simulink model "Latest_Greatest"  (Simulink 10.1)
settings: Solver=ode4  StartTime=0  StopTime=15  FixedStep=DeltaT  RelTol=1e-3  EnableMultiTasking=on
InitFcn:
  | % Bifocal Relay Mirror Spacecraft (prior to payload installation) Dynamics Simulation          TA Sands
  | clear all;close all;clc;warning off all;
  | 
  | % Simulation run parameters
  | Rate=1000;  DeltaT=1/Rate;
  | 
  | % Maneuver Parameters
  | roll=0;  pitch=0; yaw=60;   roll=roll*pi/180; pitch=pitch*pi/180; yaw=yaw*pi/180;
  | SlewTime=5;   SACengage=0;
  | 
  | %Constants0
  | Re=6371.2e3;mu=398601.2e9;          %earth radius and universal gravitation constant
  | 
  | %Spacecraft orbit
  | h=0;                                     %orbit altitude
  | R=Re+h;                             %orbit radius from center of earth
  | we=0.000072921158553;   %earth's angular velocity rad/solar sec(Vallado)
  | wo=sqrt(mu/(Re+h)^3);        %orbit angular velocity
  | incln=36.6001*pi/180;          %Inclination assumed Monterey Latitude
  | epsilon=12*pi/180;  alphao=0;
  | uo=0; nuo=0;                        %Start S/C beneath subsolar point
  | beta=60; gamma=1.5;
  | a=0.545491852; b=0.314939867;  c=0.704226952;   %Assumed spacecraft rectangular size
  | Area=[b*c a*c a*b];                 %projected area~m^2 in body x,y,z directions
  | density=4.39e-14;
  | kpre=-9.9639/24/3600/180*pi*0;      %nodal precession constant assumed zero here
  | wn=kpre*(Re/(Re+h))^3.5*cos(incln); %nodal precession (zero eccentricity)
  | V=wo*(Re+h);
  | rho=asin(Re/(h+Re));                %earth angular radius
  | Cd=2.5;     psun=4.5E-6;            %Drag coefficient and solar pressure constant~N/m^2
  | Kaero=-0.5*Cd*V^2;   Psolar=2*psun;  %constants for aero and solar torque calculation
  | dL=[0.002 0.002 0.008];             %predicted distance between cp and cg
  | Kme=2.3390e-005;
  | 
  | %Spacecraft Magnetic Properties (assumed)
  | mresid=[0 0 0.01];                  %Spacecraft residual magnetic moment
  | M=mresid;                           %Magnetic unit dipole vector
  | K=7.943e15;
  | 
  | % ACTUAL Spacecraft Inertia conditions
  | Ix=90;   Iy=100;   Iz=250 ;
  | Ixy=-10;  Iyz=20;  Ixz=-10;
  | Imo=[Ix -Ixy -Ixz;
  |        -Ixy  Iy  -Iyz;
  |        -Ixz -Iyz  Iz];                  %Moment of inertia matrix
  | Iinv=inv(Imo);                      %Moment of inertia inverse goes in dynamics block
  | 
  | %Spacecraft initial Euler state angles and rates
  | phio=0;thetao=0;psio=0;                    %Initial Euler Angles
  | phidoto=0;thetadoto=0;psidoto=0;     %Initial Euler Rates
  | 
  | %Calculation of initial quaternion (qo) and angular momentum (Ho)
  | s1=sin(phio/2);s2=sin(thetao/2);s3=sin(psio/2);c1=cos(phio/2);c2=cos(thetao/2);c3=cos(psio/2);
  | q1o=s1*c2*c3-c1*s2*s3;
  | q2o=c1*s2*c3+s1*c2*s3;              %Wie pg. 321
  | q3o=c1*c2*s3-s1*s2*c3;
  | q4o=c1*c2*c3+s1*s2*s3;
  | S1=sin(phio);S2=sin(thetao);S3=sin(psio);C1=cos(phio);C2=cos(thetao);C3=cos(psio);
  | wxo=phidoto-psidoto*S2-wo*S3*C2;
  | wyo=thetadoto*C1+psidoto*C2*S1-wo*(C3*C1+S3*S2*S1);
  | wzo=psidoto*C2*C1-thetadoto*S1-wo*(S3*S2*C1-C3*S1);
  | qo=[q1o q2o q3o q4o];
  | Ho=Imo*[wxo wyo wzo]';
  | norm(Ho)*1000;
  | 
  | %Calculate eclipse time for comparison with EPS calculations
  | Te=100.87*2*V/2/pi;
  | 
  | %CMG Properties (in degrees)
  | %beta=90*pi/180;                                     %Skew angle in degrees converted to radians
  | beta=[90;90;-90;0]; beta=beta.*pi./180;
  | %beta=[54.73;54.73;-54.73;0]; beta=beta.*pi./180;
  | 
  | Gimbal0=[-30*pi/180; 90*pi/180; -30*pi/180;0];   % Initial Gimbal angles for 0 H spin up
  | w_wheel=2800*(2*pi/60);                       %Wheel speed in RPM converted to rad/s
  | Iwheel=0.0614*1.3558179483314;        % Wheel inertia in slug-ft^2 converted (exact) to kg m^2
  | h_wheel=Iwheel*w_wheel;                     % CMG Wheel Angular Momentum
  | 
  | %FEEDFORWARD (ASSUMED) Spacecraft Inertia conditions
  | Ix=119.1259;   Iy=150.6615;   Iz=106.0288;   %ACTUAL Values are Ix=90;   Iy=100;   Iz=250 ;
  | Ixy=-15.7678;  Iyz=22.31637;  Ixz=-6.54859;  %ACTUAL Values are Ixy=-10;  Iyz=20;  Ixz=-10;
  | Imo=[Ix -Ixy -Ixz;
  |        -Ixy  Iy  -Iyz;
  |        -Ixz -Iyz  Iz];                  %Moment of inertia matrix
  | THETAo=[Ix Ixy Ixz Iy Iyz Iz 0 0 0];
  | 
  | % [Fossen]'s adaptive feedforward parameters
  | ETA=1;LAMBDA=0;  uffGain=1;
  | 
  | %FEEDBACK CONTROLLERS Follow
  | %PDI Controller Gains  % TUNED Well for Presence of LOWPASS (Kp=0.5; Kd=Kp*750;  Ki=0.1)
  | %Kp=0.5;  Kd=Kp*750;  Ki=0.1;
  | 
  | %PDI Controller Gains  % TUNED WELL FOR NO-NOISE (Kp=1; Kd=2000*Kp; Ki=5)
  | Kp=1;   Kd=Kp*6000;    Ki=5;
  | 
  | %PDI Controller Gains  % TUNED WELL FOR NOISE (Kp=1; Kd=Kp*3000; Ki=1)
  | %Kp=1;   %Kd=Kp*3000;   %Ki=1;
  | 
  | %PID Controller Gains tuned well for uff and ufb decoupling
  | Kpx=20;  Kdx=1000;  Kix=0.1;
  | 
  | %Bandpass filter pole per Bong Wie 2nd Edition pg 137-138
  | wp=10*pi/SlewTime;       % Product of pole frequency and zero frequency establishes max phase lag
  | wz=2*wp;
  | dampZ=1;  % >0 but small for good tracking..
  | dampP=dampZ;
  | % Sensor Noise Parameters
  | NoiseVariance=1e-9;             BADNoiseVariance=NoiseVariance*1e3;
  | 
  | % Observer Gains
  | MaxI=300;  lambda1=12.5  ;   lambda2=50 ;   lambda3= 200;
  | Kdo=MaxI*(lambda1+lambda2+lambda3)/10;
  | Kpo=MaxI*(lambda1*(lambda2+lambda3)+lambda2*lambda3)/10;
  | Kio=MaxI*lambda1*lambda2*lambda3/9;
StopFcn:
  | if flag==0; Hcmg=Hcmg;else;Hcmg=HcmgMP;end;
  | Hxcmg=[];Hycmg=[];Hzcmg=[];CondA=[]; CondA_MP=[];t=[]; SingPt=[];DetA=[];
  | for i=1:max(size(A));  t=[t i*DeltaT];  H=Hcmg(:,:,i); Hx=H(1,:);  Hy=H(2,:);  Hz=H(3,:);
  | detA=det(A(:,1:3,i));Hxcmg=[Hxcmg Hx];  Hycmg=[Hycmg Hy];  Hzcmg=[Hzcmg Hz];
  | CONDA=cond(A(:,:,i));
  | DetA=[DetA detA]; DetA=1./DetA;
  | CondA=[CondA CONDA];end;   %CondA=CondA./max(CondA); DetA=DetA./max(DetA);
  | Hmag=sqrt(Hxcmg.^2+Hycmg.^2+Hzcmg.^2);x=(max(t)-DeltaT);
  | 
  | InvCondA;
  | 
  | if flag==0; MaxInvCond=min(1./CondA(10*Rate+1:end));DELTA=delta;DELTAdot=deltadot;
  | else; MaxInvCond=min(1./CondA_MP(10*Rate+1:end));DELTA=delta_MP;DELTAdot=deltadot_MP;Hcmg=HcmgMP;end;
  | 
  | ERROR=(trajectory*180/pi-Euler);
  | 
  | figure(1); wdotTrajectory=[CMDTrajectory(:,1) CMDTrajectory(:,2) CMDTrajectory(:,3)];  wTrajectory=[CMDTrajectory(:,4) CMDTrajectory(:,5) CMDTrajectory(:,6)]; ThetaTrajectory=180/pi.*[trajectory(:,1) trajectory(:,2) trajectory(:,3)];
  | subplot(3,1,1); plot(t,wdotTrajectory,'linewidth',2); axis tight; grid; ylabel('\omega^d^o^t_C_M_D (deg)','fontsize',16); title('Desired Angle, Rate, Acceleration Trajectories','fontsize',16);   set(gca,'XTick',0:2:15);     set(gca,'XTickLabel',{' ',' ',' ',' ',' ',' ',' ',' ','15'});
  | subplot(3,1,2); plot(t,wTrajectory,'linewidth',2); axis tight; grid; ylabel('\omega_C_M_D (deg)','fontsize',16);set(gca,'XTick',0:2:15);     set(gca,'XTickLabel',{' ',' ',' ',' ',' ',' ',' ',' ','15'});
  | subplot(3,1,3); plot(t,ThetaTrajectory,'linewidth',2); axis tight; grid; ylabel('\theta_C_M_D (deg)','fontsize',16); xlabel('time (sec)','fontsize',16);
  | 
  | figure(2);
  | subplot(2,1,1);plot(t,Hmag,'LineWidth',3);   ylabel('|H_c_m_g|','Fontsize',16);grid;axis([0,x,0,3]); set(gca,'fontsize',16);set(gca,'XTickLabel',{' ',' ',' ',' ',' ',' ',' ',' ','15'});
  | subplot(2,1,2);plot(t,InvCondA,'linewidth',3);grid;xlabel('t(sec)','fontsize',14,'fontname','times');ylabel('Cond[A]','fontsize',14,'fontname','times');axis([0,max(t),0,21.82]); set(gca,'fontsize',16);
  | 
  | DELTA1=DELTA(1,:);DELTA2=DELTA(2,:);DELTA3=DELTA(3,:);DELTA4=DELTA(4,:);
  | DELTAdot1=DELTAdot(1,:);DELTAdot2=DELTAdot(2,:);DELTAdot3=DELTAdot(3,:);DELTAdot4=DELTAdot(4,:);
  | 
  | figure(3);subplot(4,1,1);plot(t,DELTA1,'LineWidth',3); title('Gimbal Angles','fontsize',16);ylabel('\theta_1(deg)','Fontsize',14);grid;axis tight; set(gca,'XTickLabel',{' ',' ',' ',' ',' ',' ',' ',' ','15'});set(gca,'fontsize',16);
  | subplot(4,1,2);plot(t,DELTA2,'LineWidth',3); ylabel('\theta_2(deg)','Fontsize',16);grid;axis tight; set(gca,'XTickLabel',{' ',' ',' ',' ',' ',' ',' ',' ','15'});set(gca,'fontsize',16);
  | subplot(4,1,3);plot(t,DELTA3,'LineWidth',3); ylabel('\theta_3(deg)','Fontsize',16);grid;axis tight; set(gca,'XTickLabel',{' ',' ',' ',' ',' ',' ',' ',' ','15'});set(gca,'fontsize',16);
  | subplot(4,1,4);plot(t,InvCondA,'linewidth',3);grid;xlabel('t(sec)','fontsize',14,'fontname','times');ylabel('Cond[A]','fontsize',14,'fontname','times');axis([0,max(t),0,21.82]); set(gca,'fontsize',16);
  | 
  | figure(4);subplot(4,1,1);plot(t,DELTAdot1,'LineWidth',3);  title('Gimbal Angle RATES','fontsize',16); ylabel('\theta_d_o_t_1(rad/s)','Fontsize',16);grid; axis([0,x,-pi*1.1,pi*1.1]);   set(gca,'XTickLabel',{' ',' ',' ',' ',' ',' ',' ',' ','15'});set(gca,'fontsize',16);
  | subplot(4,1,2);plot(t,DELTAdot2,'LineWidth',3);   ylabel('\theta_d_o_t_2(rad/s)','Fontsize',16);grid;axis([0,x,-pi*1.1,pi*1.1]);   set(gca,'XTickLabel',{' ',' ',' ',' ',' ',' ',' ',' ','15'});   set(gca,'fontsize',16);
  | subplot(4,1,3);plot(t,DELTAdot3,'LineWidth',3);   ylabel('\theta_d_o_t_3(rad/s)','Fontsize',16);grid;axis([0,x,-pi*1.1,pi*1.1]); set(gca,'XTickLabel',{' ',' ',' ',' ',' ',' ',' ',' ','15'});set(gca,'fontsize',16);
  | subplot(4,1,4);plot(t,InvCondA,'linewidth',3);grid;xlabel('t(sec)','fontsize',14,'fontname','times');ylabel('Cond[A]','fontsize',14,'fontname','times');axis([0,max(t),0,21.82]); set(gca,'fontsize',16);
  | 
  | figure(5);
  | subplot(4,1,1);plot(t,Hxcmg,'linewidth',3);axis([0,x,-3.25,3.25]);grid;ylabel('h_x/|h|','fontsize',16);title('Normalized Momentum','fontsize',16);set(gca,'XTickLabel',{' ',' ',' ',' ',' ',' ',' ',' ','15'});set(gca,'fontsize',16);
  | subplot(4,1,2);plot(t,Hycmg,'linewidth',3);axis([0,x,-3.25,3.25]);grid;ylabel('h_y/|h|','fontsize',16);set(gca,'XTickLabel',{' ',' ',' ',' ',' ',' ',' ',' ','15'});set(gca,'fontsize',16);
  | subplot(4,1,3);plot(t,Hzcmg,'linewidth',3);axis([0,x,-3.25,3.25]);grid;ylabel('h_z/|h|','fontsize',16);  set(gca,'XTickLabel',{' ',' ',' ',' ',' ',' ',' ',' ','15'});set(gca,'fontsize',16);
  | subplot(4,1,4);plot(t,InvCondA,'linewidth',3);grid;xlabel('t(sec)','fontsize',14,'fontname','times');ylabel('Cond[A]','fontsize',14,'fontname','times');axis([0,max(t),0,21.82]); set(gca,'fontsize',16);
  | 
  | figure(6); EulerX=Euler(:,1);EulerY=Euler(:,2);EulerZ=Euler(:,3);
  | subplot(4,1,1);plot(t,EulerX,'linewidth',3); axis([0,x,min(EulerX)*5,max(EulerX)*5]);grid;ylabel('\phi(deg)','fontsize',16);title('True Euler Angles','fontsize',14);  set(gca,'XTickLabel',{' ',' ',' ',' ',' ',' ',' ',' ','15'});  set(gca,'fontsize',16);
  | subplot(4,1,2);plot(t,EulerY,'linewidth',3);  axis([0,x,min(EulerY)*5,max(EulerY)*5]); grid;ylabel('\theta(deg)','fontsize',14);  set(gca,'XTickLabel',{' ',' ',' ',' ',' ',' ',' ',' ','15'}); set(gca,'fontsize',16);
  | subplot(4,1,3);plot(t,EulerZ,'linewidth',3);axis([0,x,min(EulerZ)*1.25,max(EulerZ)*1.25]);grid;  ylabel('\psi(deg)','fontsize',14);  set(gca,'XTickLabel',{' ',' ',' ',' ',' ',' ',' ',' ','15'});  set(gca,'fontsize',16);
  | subplot(4,1,4);plot(t,InvCondA,'linewidth',3);grid;xlabel('t(sec)','fontsize',14,'fontname','times');ylabel('Cond[A]','fontsize',14,'fontname','times');axis([0,max(t),0,21.82]); set(gca,'fontsize',16);
  | 
  | EX=ERROR(:,1);  EY=ERROR(:,2);     EZ=ERROR(:,3);
  | MeanXerror=mean(EX); Xmean=num2str(MeanXerror); xmean=['\mu_\phi=', Xmean];
  | STDx=std(EX);Xsigma=num2str(STDx);SigmaX=['    \sigma_x=' Xsigma];  xlegend=[xmean, SigmaX];
  | MeanYerror=mean(EY); Ymean=num2str(MeanYerror); ymean=['\mu_\theta=', Ymean];
  | STDy=std(EY); Ysigma=num2str(STDy);SigmaY=['    \sigma_y=' Ysigma]; ylegend=[ymean, SigmaY];
  | MeanZerror=mean(EZ); Zmean=num2str(MeanZerror); zmean=['\mu_\psi=', Zmean];
  | STDz=std(EZ);Zsigma=num2str(STDz);SigmaZ=['    \sigma_z=' Zsigma]; zlegend=[zmean, SigmaZ];
  | MeanError=[MeanXerror MeanYerror MeanZerror];  StdDev=[STDx STDy STDz];
  | 
  | figure(7);
  | subplot(3,1,1);plot(t,EX,'linewidth',3);    axis([0,x,min(EX)*1.25,max(EX)*1.25]);  title('Euler Angle Tracking Error','fontsize',16);
  |      legend(xlegend, 'location','NorthEast');  grid   ; ylabel('\phi(deg)','fontsize',16);set(gca,'XTickLabel',{' ',' ',' ',' ',' ',' ',' ',' ','15'});set(gca,'fontsize',16);
  | subplot(3,1,2);plot(t,EY,'linewidth',3);   axis([0,x,min(EY)*1.25,max(EY)*1.25]);
  |       legend(ylegend, 'location','NorthEast');  grid;    ylabel('\theta(deg)','fontsize',16);set(gca,'XTickLabel',{' ',' ',' ',' ',' ',' ',' ',' ','15'});set(gca,'fontsize',16);
  | subplot(3,1,3);plot(t,EZ,'linewidth',3);    axis([0,x,min(EZ)*1.25,max(EZ)*1.25]);
  |      legend(zlegend, 'location','NorthEast');  grid;   ylabel('\psi(deg)','fontsize',16);xlabel('t(sec)','fontsize',16);set(gca,'fontsize',16);
  | 
  | figure(8);subplot(3,3,1);
  | plot(t,THETAhat(:,1),'linewidth',2);grid; axis tight;ylabel('J_x_x','fontsize',16);  set(gca,'XTickLabel',{' ',' ',' ',' ',' ',' ',' ',' ','15'});  set(gca,'fontsize',16);
  | subplot(3,3,2);plot(t,THETAhat(:,2),'linewidth',3);grid;axis tight;ylabel('J_x_y','fontsize',16);   set(gca,'XTickLabel',{' ',' ',' ',' ',' ',' ',' ',' ','15'});  set(gca,'fontsize',16);  title('Inertia & Momentum Adaption','fontsize',18);
  | subplot(3,3,3);plot(t,THETAhat(:,3),'linewidth',3);grid;axis tight;ylabel('J_x_z','fontsize',16);set(gca,'XTickLabel',{' ',' ',' ',' ',' ',' ',' ',' ','15'});set(gca,'fontsize',16);
  | subplot(3,3,4);plot(t,THETAhat(:,4),'linewidth',3);grid;axis tight;ylabel('J_y_y','fontsize',16);set(gca,'XTickLabel',{' ',' ',' ',' ',' ',' ',' ',' ','15'});set(gca,'fontsize',16);
  | subplot(3,3,5);plot(t,THETAhat(:,5),'linewidth',3);grid;axis tight;ylabel('J_y_z','fontsize',16);set(gca,'XTickLabel',{' ',' ',' ',' ',' ',' ',' ',' ','15'});set(gca,'fontsize',16);
  | subplot(3,3,6);plot(t,THETAhat(:,6),'linewidth',3);grid;axis tight;ylabel('J_z_z','fontsize',16);set(gca,'XTickLabel',{' ',' ',' ',' ',' ',' ',' ',' ','15'});set(gca,'fontsize',16);
  | subplot(3,3,7);plot(t,THETAhat(:,7),'linewidth',3);grid;axis tight;ylabel('H_x','fontsize',16);xlabel('t(sec)','fontsize',14);set(gca,'fontsize',16);
  | subplot(3,3,8);plot(t,THETAhat(:,8),'linewidth',3);grid;axis tight;ylabel('H_y','fontsize',16);xlabel('t(sec)','fontsize',14);set(gca,'fontsize',16);
  | subplot(3,3,9);plot(t,THETAhat(:,9),'linewidth',3);grid;axis tight;ylabel('H_z','fontsize',16);xlabel('t(sec)','fontsize',14);set(gca,'fontsize',16);
  | 
  | ControlX=sqrt(abs(ControlEffort(end,1)))/(max(t)); ControlStringX=num2str(ControlX); Control_x=['1/t sqrt(\int u^2_\phi dt)=', ControlStringX];
  | ControlY=sqrt(abs(ControlEffort(end,2)))/(max(t)); ControlStringY=num2str(ControlY); Control_y=['1/t sqrt(\int u^2_\theta dt)=', ControlStringY];
  | ControlZ=sqrt(abs(ControlEffort(end,3)))/(max(t)); ControlStringZ=num2str(ControlZ); Control_z=['1/t sqrt(\int u^2_\psi dt)=', ControlStringZ];
  | 
  | figure(9);
  | subplot(2,1,1);plot(t,ufb,'linewidth',3);grid; axis tight;ylabel('Feedback Control (Nm)','fontname','times','fontsize',14);  legend(Control_x, Control_y, Control_z, 'location','SouthEast');
  | title('Feedforward and Feedback Controls','fontsize',18);set(gca,'XTickLabel',{' ',' ',' ',' ',' ',' ',' ',' ','15'});set(gca,'fontsize',16);
  | subplot(2,1,2);plot(t,uff,'linewidth',3);grid; axis tight; ylabel('FeedForward Control (Nm)','fontname','times','fontsize',14);      xlabel('time(sec)','fontname','times','fontsize',14); set(gca,'fontsize',16);
  | 
  | figure(10);
  | subplot(4,1,1);plot(t,ufb(:,1),'linewidth',3);grid;ylabel('u_\phi(Nm)','fontsize',16);title('u_f_b (Nm)','fontsize',16); axis tight; set(gca,'XTickLabel',{' ',' ',' ',' ',' ',' ',' ',' ','15'});set(gca,'fontsize',16);
  | subplot(4,1,2);plot(t,ufb(:,2),'linewidth',3); grid;ylabel('u_\theta(Nm)','fontsize',16); axis tight; set(gca,'XTickLabel',{' ',' ',' ',' ',' ',' ',' ',' ','15'});set(gca,'fontsize',16);
  | subplot(4,1,3);plot(t,ufb(:,3),'linewidth',3); grid;ylabel('u_\psi(Nm)','fontsize',16); axis tight; set(gca,'XTickLabel',{' ',' ',' ',' ',' ',' ',' ',' ','15'});set(gca,'fontsize',16);
  | subplot(4,1,4);plot(t,InvCondA,'linewidth',3);grid;xlabel('t(sec)','fontsize',14,'fontname','times');ylabel('Cond[A]','fontsize',14,'fontname','times');axis([0,max(t),0,21.82]); set(gca,'fontsize',16);
  | 
  | % CALCULATE FIGURES OF MERIT FOR ESTIMATION ACCURACY OF LUENBERGER OBSERVER
  | EEX=EstimationError(:,1);EEY=EstimationError(:,2);EEZ=EstimationError(:,3);
  | MeanEEX=mean(EEX); EEXmean=num2str(MeanEEX); Exmean=['Luenberger \mu_\phi^o _E_r_r_o_r=', EEXmean];
  | MeanEEY=mean(EEY); EEYmean=num2str(MeanEEY); Eymean=['Luenberger \mu_\theta^o _E_r_r_o_r=', EEYmean];
  | MeanEEZ=mean(EEZ); EEZmean=num2str(MeanEEZ); Ezmean=['Luenberger \mu_\psi^o _E_r_r_o_r=', EEZmean];
  | STDEEX=std(EEX);                      EEXstd=num2str(STDEEX);         Exstd=['   \sigma_\phi^o _E_r_r_o_r=', EEXstd];
  | STDEEY=std(EEY);                      EEYstd=num2str(STDEEY);         Eystd=['   \sigma_\theta^o _E_r_r_o_r=', EEYstd];
  | STDEEZ=std(EEZ);                      EEZstd=num2str(STDEEZ);         Ezstd=['   \sigma_\psi^o _E_r_r_o_r=', EEZstd];
  | XlabelLuen=[Exmean Exstd];  YlabelLuen=[Eymean Eystd];  ZlabelLuen=[Ezmean Ezstd];
  | 
  | % CALCULATE FIGURES OF MERIT FOR ESTIMATION ACCURACY OF PID OBSERVERS
  | EEXo=PIDoEstimationError(:,1);EEYo=PIDoEstimationError(:,2);EEZo=PIDoEstimationError(:,3);
  | MeanEEXo=mean(EEXo); EEXmeano=num2str(MeanEEXo); Exmeano=['PID \mu_\phi^o _E_r_r_o_r=', EEXmeano];
  | MeanEEYo=mean(EEYo); EEYmeano=num2str(MeanEEYo); Eymeano=['PID \mu_\theta^o _E_r_r_o_r=', EEYmeano];
  | MeanEEZo=mean(EEZo); EEZmeano=num2str(MeanEEZo); Ezmeano=['PID \mu_\psi^o _E_r_r_o_r=', EEZmeano];
  | STDEEXo=std(EEXo);                      EEXstdo=num2str(STDEEXo);         Exstdo=['    \sigma_\phi^o _E_r_r_o_r=', EEXstdo];
  | STDEEYo=std(EEYo);                      EEYstdo=num2str(STDEEYo);         Eystdo=['    \sigma_\theta^o _E_r_r_o_r=', EEYstdo];
  | STDEEZo=std(EEZo);                      EEZstdo=num2str(STDEEZo);         Ezstdo=['    \sigma_\psi^o _E_r_r_o_r=', EEZstdo];
  | XlabelPID=[Exmeano Exstdo];  YlabelPID=[Eymeano Eystdo];  ZlabelPID=[Ezmeano Ezstdo];
  | 
  | % CALCULATE FIGURES OF MERIT FOR ESTIMATION ACCURACY OF KALMAN OBSERVERS
  | EEXkf=KalmanEstimationError(:,1);   EEYkf=KalmanEstimationError(:,2);        EEZkf=KalmanEstimationError(:,3);
  | MeanEEXkf=mean(EEXkf);                EEXmeankf=num2str(MeanEEXkf);         Exmeankf=['Kalman \mu_\phi^o _E_r_r_o_r=', EEXmeankf];
  | MeanEEYkf=mean(EEYkf);                EEYmeankf=num2str(MeanEEYkf);         Eymeankf=['Kalman \mu_\theta^o _E_r_r_o_r=', EEYmeankf];
  | MeanEEZkf=mean(EEZkf);                EEZmeankf=num2str(MeanEEZkf);         Ezmeankf=['Kalman \mu_\psi^o _E_r_r_o_r=', EEZmeankf];
  | STDEEXkf=std(EEXkf);                      EEXstdkf=num2str(STDEEXkf);         Exstdkf=['    \sigma_\phi^o _E_r_r_o_r=', EEXstdkf];
  | STDEEYkf=std(EEYkf);                      EEYstdkf=num2str(STDEEYkf);         Eystdkf=['    \sigma_\theta^o _E_r_r_o_r=', EEYstdkf];
  | STDEEZkf=std(EEZkf);                      EEZstdkf=num2str(STDEEZkf);         Ezstdkf=['    \sigma_\psi^o _E_r_r_o_r=', EEZstdkf];
  | Xlabelkf=[Exmeankf Exstdkf];  Ylabelkf=[Eymeankf Eystdkf];  Zlabelkf=[Ezmeankf Ezstdkf];
  | 
  | figure(11);
  | subplot(3,1,1);plot(t,KalmanEstimationError(:,1),'r:','linewidth',3); hold on; plot(t,PIDoEstimationError(:,1),'linewidth',3);  plot(t,EstimationError(:,1),'k--','linewidth',3);   set(gca,'fontsize',12);
  | ylabel('\phi Roll (deg)','fontsize',16);   title('Observer Estimation Error Comparison','fontsize',14);  legend(Xlabelkf,XlabelPID, XlabelLuen, 'location','NorthWest'); grid; axis([0,15,-0.01,0.04]);
  | set(gca,'XTickLabel',{' ',' ',' ',' ',' ',' ',' ',' ','15'});
  | 
  | subplot(3,1,2); plot(t,KalmanEstimationError(:,2),'r:','linewidth',3); hold on;  plot(t,PIDoEstimationError(:,2),'linewidth',3); plot(t,EstimationError(:,2),'k--','linewidth',3); set(gca,'fontsize',12);
  | ylabel('\theta Pitch (deg)','fontsize',16); hold off;  legend(Ylabelkf, YlabelPID, YlabelLuen, 'location','SouthWest'); grid;  set(gca,'XTickLabel',{' ',' ',' ',' ',' ',' ',' ',' ','15'});  axis([0,15,-0.08,0.03]);
  | 
  | subplot(3,1,3); plot(t,KalmanEstimationError(:,3),'r:','linewidth',3);  hold on;  plot(t,PIDoEstimationError(:,3),'linewidth',3);plot(t,EstimationError(:,3),'k--','linewidth',3);set(gca,'fontsize',12);
  | ylabel('\psi Yaw (deg)','fontsize',16);xlabel('t(sec)','fontsize',16);  hold off;  legend(Zlabelkf, ZlabelPID, ZlabelLuen,'location','NorthWest'); grid; axis tight;
  | 
  | %openfig('90_Degree_Singularity_Hypersurface');hold on;plot3(Hcmg(1,:),Hcmg(2,:),Hcmg(3,:), 'LineWidth',3);hold off;
  | 
  | QNORMSTD=std(qnorm);                      QNORMSTDSTRING=num2str(QNORMSTD);         QnormLEGEND=['    ||q||=', QNORMSTDSTRING];
  |  figure (12); plot(qnorm); legend([QnormLEGEND]);  grid;
undefined symbols (not defined in the file): magnitude, svd
libraries: aerospace x3, simulink_need_slupdate x2, dspadpt3 x2, dspinverses x1
(part 1 of 2)
settings Model: Creator=tasands  LastModifiedBy=Cornell Gaming Lapto
settings DataIOCC: LimitDataPoints=on  SignalLoggingSaveFormat=ModelDataLogs  SignalLoggingName=sigsOut
settings OptimizationCC: ExpressionDepthLimit=2147483647  InitFltsAndDblsToZero=on
settings DebuggingCC: SaveWithParameterizedLinksMsg=none  SignalResolutionControl=TryResolveAllWithWarning  MultiTaskDSMMsg=warning  MultiTaskCondExecSysMsg=none  FcnCallInpInsideContextMsg=warning  StateNameClashWarn=warning  PregeneratedLibrarySubsystemCodeDiagnostic=none
settings HardwareCC: TargetHWDeviceType=32-bit Generic  ProdEqTarget=off
settings GRTTargetCC: TargetFcnLib=ansi_tfl_tmw.mat

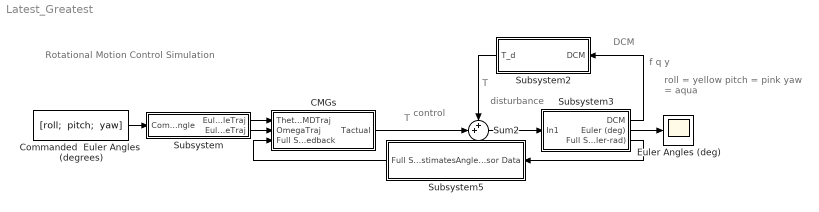
== system Latest_Greatest ==
  note: roll = yellow
      | pitch = pink
      | yaw = aqua
  note: Rotational Motion Control Simulation
  note: f
      | q
      | y
  note: T
  note: disturbance
  note: T
  note: control
  note: DCM
  CMGs : Subsystem
      mask Display: disp('Actuators & Control')
  "Commanded  Euler Angles  (degrees) " : Constant  Value="[roll;  pitch;  yaw]"
  Euler Angles (deg) : Scope
      settings: StartFcn=|
      | %Simulink figure properties
      | shh=get(0,'ShowHiddenHandles');
      | set(0,'ShowHiddenHandles','On')
      | set(gcf,'menubar','figure')
      | set(gcf,'CloseRequestFcn','closereq')
      | set(gcf,'DefaultLineClipping','Off')
      | set(0,'ShowHiddenHandles',shh)
      | %set(gca,'LineWidth',3)
  Subsystem : Subsystem
      mask Display: disp('Generate Trajectory')
  Subsystem2 : Subsystem
      mask Display: disp('Disturbances')
  Subsystem3 : Subsystem
      mask Display: disp('Dynamics')
  Subsystem5 : Subsystem
      mask Display: disp('Sensors & Observers')
  Sum2 : Sum  Inputs=++|  SaturateOnIntegerOverflow=on
  wires:
  Sum2/1 -> Subsystem3/1(In1)
  CMGs/1(Tactual) -> Sum2/2
  Subsystem3/2(Euler (deg)) -> Euler Angles (deg)/1
  Subsystem2/1(T_d) -> Sum2/1
  "Commanded  Euler Angles  (degrees) "/1 -> Subsystem/1(Commanded Euler Angle)
  Subsystem3/1(DCM) -> Subsystem2/1(DCM)
  Subsystem/1(EulerAngleTraj) -> CMGs/1(ThetaCMDTraj)
  Subsystem5/1(Full State Estimates) -> CMGs/3(Full State Feedback)
  Subsystem3/3(Full State  Feedback  (Euler-rad)) -> Subsystem5/1(Angle & Rate  Sensor Data)
  Subsystem/2(EulerRateTraj) -> CMGs/2(OmegaTraj)

== system Latest_Greatest/CMGs ==
  note: TA Sands
  note: Controller & Actuators
  note: HOMOGENEOUS SOLUTION (INITIAL CONDITIONS)
      | NOT TOTALLY DECOUPLED IN CONTROL (theta double dot)
  ThetaCMDTraj : Inport
  OmegaTraj : Inport  Port=2
  Full State Feedback : Inport  Port=3
  CMG Steering Logic1 : Subsystem
      mask Display: disp('CMG Steering & Decoupling')
  Subsystem1 : Subsystem
      mask Display: disp('displays & scopes')
  Subsystem3 : Subsystem
      mask Display: disp('Controllers')
  Tactual : Outport  VectorParamsAs1DForOutWhenUnconnected=off
  wires:
  Full State Feedback/1 -> Subsystem3/3(FullStateFeedback)
  ThetaCMDTraj/1 -> Subsystem3/1(ThetaCMDTraj)
  Subsystem3/2(u) -> Subsystem1/3(In2), CMG Steering Logic1/2(u)
  Subsystem1/1(Out1) -> Tactual/1
  CMG Steering Logic1/1(Tc) -> Subsystem1/1(In1)
  CMG Steering Logic1/2(d) -> Subsystem1/2(In3)
  Subsystem3/1(w) -> CMG Steering Logic1/1(w)
  OmegaTraj/1 -> Subsystem3/2(OmegaCMDTraj)

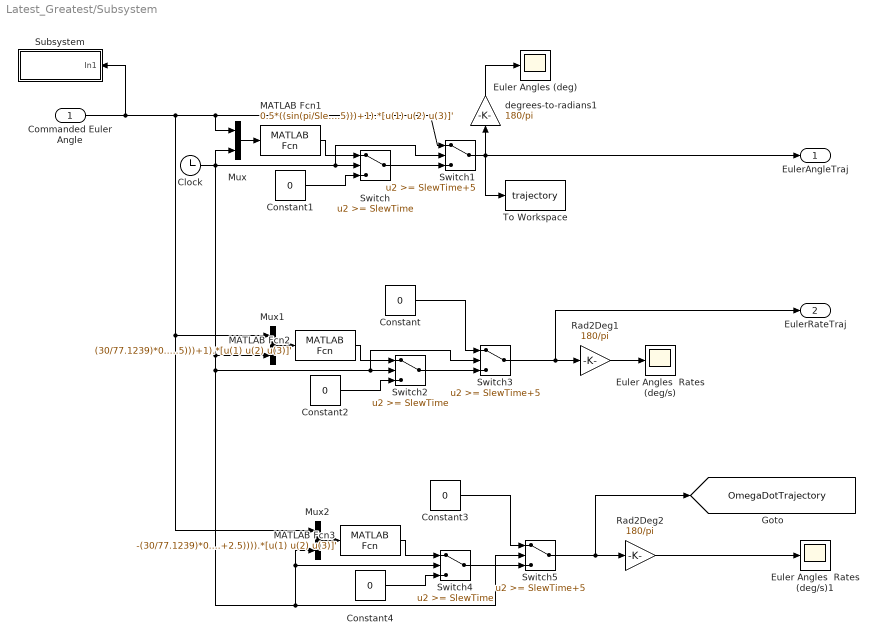
== system Latest_Greatest/Subsystem ==
  Commanded Euler Angle : Inport
  Clock : Clock
  Constant{,1..4} (5 alike) : Constant  Value=0
  Euler Angles (deg) : Scope
      settings: StopFcn=|
      | %Simulink figure properties
      | shh=get(0,'ShowHiddenHandles');
      | set(0,'ShowHiddenHandles','On')
      | set(gcf,'menubar','figure')
      | set(gcf,'CloseRequestFcn','closereq')
      | set(gcf,'DefaultLineClipping','Off')
      | set(0,'ShowHiddenHandles',shh)
  Euler Angles  Rates (deg/s) : Scope
      settings: StopFcn=|
      | %Simulink figure properties
      | shh=get(0,'ShowHiddenHandles');
      | set(0,'ShowHiddenHandles','On')
      | set(gcf,'menubar','figure')
      | set(gcf,'CloseRequestFcn','closereq')
      | set(gcf,'DefaultLineClipping','Off')
      | set(0,'ShowHiddenHandles',shh)
  Euler Angles  Rates (deg/s)1 : Scope
      settings: StopFcn=|
      | %Simulink figure properties
      | shh=get(0,'ShowHiddenHandles');
      | set(0,'ShowHiddenHandles','On')
      | set(gcf,'menubar','figure')
      | set(gcf,'CloseRequestFcn','closereq')
      | set(gcf,'DefaultLineClipping','Off')
      | set(0,'ShowHiddenHandles',shh)
  MATLAB Fcn1 : MATLABFcn  MATLABFcn=0.5*((sin(pi/SlewTime*(u(4)+2.5)))+1).*[u(1) u(2) u(3)]'
  MATLAB Fcn2 : MATLABFcn  MATLABFcn=(30/77.1239)*0.5*(pi/SlewTime)*((cos(pi/SlewTime*(u(4)+2.5)))+1).*[u(1) u(2) u(3)]'
  MATLAB Fcn3 : MATLABFcn  MATLABFcn=-(30/77.1239)*0.5*(pi/SlewTime)^(2)*((sin(pi/SlewTime*(u(4)+2.5)))).*[u(1) u(2) u(3)]'
  Mux : Mux  Inputs=2
  Mux1 : Mux  Inputs=2
  Mux2 : Mux  Inputs=2
  Rad2Deg1 : Gain  Gain=180/pi
  Rad2Deg2 : Gain  Gain=180/pi
  Subsystem : Subsystem
      mask Display: disp('To Workspace')
  Switch : Switch  Threshold=SlewTime
  Switch1 : Switch  Threshold=SlewTime+5
  Switch2 : Switch  Threshold=SlewTime
  Switch3 : Switch  Threshold=SlewTime+5
  Switch4 : Switch  Threshold=SlewTime
  Switch5 : Switch  Threshold=SlewTime+5
  To Workspace : ToWorkspace  VariableName=trajectory  SampleTime=-1
  degrees-to-radians1 : Gain  Gain=180/pi
  EulerAngleTraj : Outport  VectorParamsAs1DForOutWhenUnconnected=off
  EulerRateTraj : Outport  Port=2  VectorParamsAs1DForOutWhenUnconnected=off
  tag scope: OmegaDotTrajectory=global
  wires:
  Switch1/1 -> EulerAngleTraj/1, To Workspace/1, degrees-to-radians1/1
  Switch/1 -> Switch1/3
  Constant1/1 -> Switch/3
  Clock/1 -> Switch/2, Switch1/2, Mux/2, Mux1/2, Switch3/2, Switch2/2, Mux2/2, Switch4/2, Switch5/2
  MATLAB Fcn1/1 -> Switch/1
  Commanded Euler Angle/1 -> Subsystem/1(In1), Mux/1, Switch1/1, Mux1/1, Mux2/1
  Mux/1 -> MATLAB Fcn1/1
  degrees-to-radians1/1 -> Euler Angles (deg)/1
  Rad2Deg1/1 -> Euler Angles  Rates (deg/s)/1
  Mux1/1 -> MATLAB Fcn2/1
  MATLAB Fcn2/1 -> Switch2/1
  Constant2/1 -> Switch2/3
  Switch2/1 -> Switch3/3
  Constant/1 -> Switch3/1
  Switch3/1 -> Rad2Deg1/1, EulerRateTraj/1
  Switch5/1 -> Rad2Deg2/1, [OmegaDotTrajectory]
  Constant3/1 -> Switch5/1
  Switch4/1 -> Switch5/3
  Constant4/1 -> Switch4/3
  MATLAB Fcn3/1 -> Switch4/1
  Mux2/1 -> MATLAB Fcn3/1
  Rad2Deg2/1 -> Euler Angles  Rates (deg/s)1/1

== system Latest_Greatest/Subsystem2 ==
  DCM : Inport
  Sum2 : Sum  Inputs=++|  SaturateOnIntegerOverflow=on
  Tdisturbance : Step  Time=0  After=0  SampleTime=0
  Tgg : Subsystem
      mask Display: disp('CG offet')
  T_d : Outport  VectorParamsAs1DForOutWhenUnconnected=off
  wires:
  Tdisturbance/1 -> Sum2/1
  Tgg/1(Tgg) -> Sum2/2
  Sum2/1 -> T_d/1
  DCM/1 -> Tgg/1(DCM)

== system Latest_Greatest/Subsystem3 ==
  note: w
  note: N B
  In1 : Inport
  Body  Dynamics : Subsystem
      mask Display: disp('Kinetics')
  Euler RATES (deg/s) : Scope
      settings: StopFcn=|
      | %Simulink figure properties
      | shh=get(0,'ShowHiddenHandles');
      | set(0,'ShowHiddenHandles','On')
      | set(gcf,'menubar','figure')
      | set(gcf,'CloseRequestFcn','closereq')
      | set(gcf,'DefaultLineClipping','Off')
      | set(0,'ShowHiddenHandles',shh)
  Mux : Mux  Inputs=2
  Subsystem1 : Subsystem
      mask Display: disp('Kinematics')
  DCM : Outport  VectorParamsAs1DForOutWhenUnconnected=off
  Euler (deg) : Outport  Port=2  VectorParamsAs1DForOutWhenUnconnected=off
  Full State  Feedback  (Euler-rad) : Outport  Port=3  VectorParamsAs1DForOutWhenUnconnected=off
  tag scope: ActualEuler=global
  wires:
  Body  Dynamics/1(NwB) -> Mux/2, Euler RATES (deg/s)/1, Subsystem1/1(wbn)
  Subsystem1/1(DCM) -> DCM/1
  In1/1 -> Body  Dynamics/1(T)
  Subsystem1/2(Euler(deg)) -> Euler (deg)/1, [ActualEuler]
  Subsystem1/3(Euler(rad)) -> Mux/1
  Mux/1 -> Full State  Feedback  (Euler-rad)/1

== system Latest_Greatest/Subsystem5 ==
  note: FULL STATE FEEDBACK (IDEAL)
  note: FULL STATE FEEDBACK (SENSOR)
  Angle & Rate  Sensor Data : Inport
  Manual Switch : ManualSwitch
  Manual Switch1 : ManualSwitch  CurrentSetting=0
  Manual Switch2 : ManualSwitch  CurrentSetting=0
  Manual Switch3 : ManualSwitch
  Manual Switch4 : ManualSwitch
  OBSERVERS (MASK THIS SUBSYSTEM AS CLASS DEMO)1 : Subsystem
      mask Display: disp('Observer')
  Subsystem2 : Subsystem
      mask Display: disp('Sensor')
  Subsystem4 : Subsystem
      mask Display: disp('Kalman Filter')
  Subsystem5 : Subsystem
      mask Display: disp('Lowpass Filter')
  Full State Estimates : Outport  VectorParamsAs1DForOutWhenUnconnected=off
  wires:
  Angle & Rate  Sensor Data/1 -> Manual Switch3/1, Subsystem2/1(Full State Feedback)
  Subsystem4/1(Out1) -> Manual Switch1/1
  Manual Switch1/1 -> Manual Switch/2
  Manual Switch2/1 -> Subsystem4/1(Full State Feedback)
  OBSERVERS (MASK THIS SUBSYSTEM AS CLASS DEMO)1/1(Estimated full state feedback (Euler-rad)) -> Manual Switch1/2, Manual Switch2/2
  Manual Switch3/1 -> Manual Switch/1
  Manual Switch4/1 -> Full State Estimates/1
  Manual Switch/1 -> Manual Switch4/1, Subsystem5/1(u)
  Subsystem2/1(Noisy  State Feedback) -> Manual Switch2/1, Manual Switch3/2, OBSERVERS (MASK THIS SUBSYSTEM AS CLASS DEMO)1/1(Full State Feedback)
  Subsystem5/1(u(filtered)) -> Manual Switch4/2

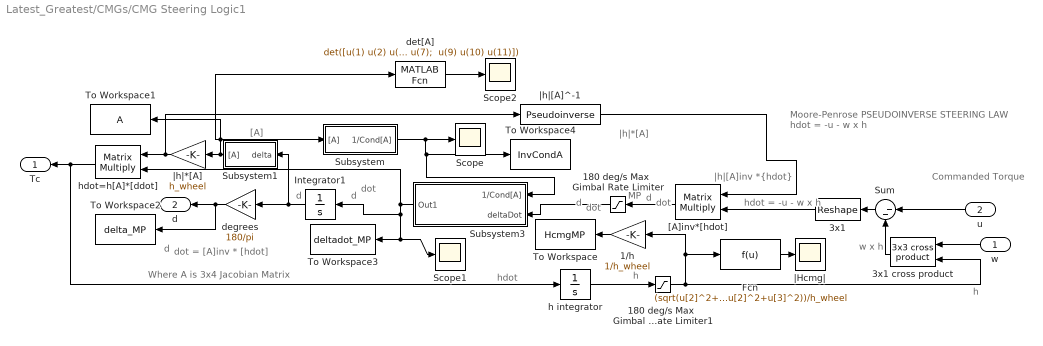
== system Latest_Greatest/CMGs/CMG Steering Logic1 ==
  note: MP
  note: d
  note: dot
  note: d
  note: [A]
  note: |h|*[A]
  note: h
  note: dot
  note: d
  note: |h|[A]inv *{hdot}
  note: Commanded
      | Torque
  note: Where A is 3x4 Jacobian Matrix
  note: d
  note: dot = [A]inv * [hdot]
  note: Moore-Penrose
      | PSEUDOINVERSE STEERING LAW
      | hdot = -u - w x h
  note: w x h
  note: dot
  note: d
  note: hdot = -u - w x h
  note: h
  note: hdot
  w : Inport
  u : Inport  Port=2
  1/h : Gain  Gain=1/h_wheel
  180 deg/s Max  Gimbal Rate Limiter : Saturate  UpperLimit=pi  LowerLimit=-pi
  180 deg/s Max  Gimbal Rate Limiter1 : Saturate  UpperLimit=[h_wheel;2*h_wheel;3*h_wheel]  LowerLimit=-1
  3x1 : Reshape  OutputDimensionality=Customize  OutputDimensions=[3,1]
  3x1 cross product : aerospace/Axes Transformations/3x3 cross product
      settings: SourceProductBaseCode=SL
  Fcn : Fcn  Expr=(sqrt(u[2]^2+u[2]^2+u[3]^2))/h_wheel
  Integrator1 : Integrator  InitialCondition=Gimbal0
  Scope : Scope
  Scope1 : Scope
  Scope2 : Scope
  Subsystem : Subsystem
      mask Display: disp('1/Cond[A]')
  Subsystem1 : Subsystem
      mask Display: disp('[A] Matrix')
  Subsystem3 : Subsystem
      mask Display: disp('SPUD')
  Sum : Sum  Inputs=|--  SaturateOnIntegerOverflow=on
  To Workspace : ToWorkspace  VariableName=HcmgMP  SampleTime=-1
  To Workspace1 : ToWorkspace  VariableName=A  SampleTime=-1
  To Workspace2 : ToWorkspace  VariableName=delta_MP  SampleTime=-1
  To Workspace3 : ToWorkspace  VariableName=deltadot_MP  SampleTime=-1
  To Workspace4 : ToWorkspace  VariableName=InvCondA  SampleTime=-1
  "[A]inv*[hdot]" : Product  Multiplication=Matrix(*)  SaturateOnIntegerOverflow=on  OutDataTypeStr=Inherit: Same as first input
  degrees : Gain  Gain=180/pi
  det[A] : MATLABFcn  MATLABFcn="det([u(1) u(2) u(3);  u(5) u(6) u(7);  u(9) u(10) u(11)])"
  h integrator : Integrator
  hdot=h[A]*[ddot] : Product  Multiplication=Matrix(*)  SaturateOnIntegerOverflow=on  OutDataTypeStr=Inherit: Same as first input
  |Hcmg| : Scope
  |h|*[A] : Gain  Gain=h_wheel
  |h|[A]^-1 : dspinverses/Pseudoinverse  wanterr=off  SimulateUsing=Interpreted execution
      settings: SourceProductBaseCode=DS
  Tc : Outport  VectorParamsAs1DForOutWhenUnconnected=off
  d : Outport  Port=2  VectorParamsAs1DForOutWhenUnconnected=off
  wires:
  Subsystem3/1(Out1) -> Integrator1/1, To Workspace3/1, Scope1/1, hdot=h[A]*[ddot]/2
  180 deg/s Max  Gimbal Rate Limiter/1 -> Subsystem3/2(deltaDot)
  degrees/1 -> To Workspace2/1, d/1
  Integrator1/1 -> degrees/1, Subsystem1/1(delta)
  Subsystem1/1("[A]") -> det[A]/1, To Workspace1/1, Subsystem/1("[A]"), |h|*[A]/1
  Fcn/1 -> |Hcmg|/1
  "[A]inv*[hdot]"/1 -> 180 deg/s Max  Gimbal Rate Limiter/1
  180 deg/s Max  Gimbal Rate Limiter1/1 -> 3x1 cross product/2, 1/h/1, Fcn/1
  3x1/1 -> "[A]inv*[hdot]"/2
  |h|*[A]/1 -> |h|[A]^-1/1, hdot=h[A]*[ddot]/1
  hdot=h[A]*[ddot]/1 -> h integrator/1, Tc/1
  u/1 -> Sum/1
  Sum/1 -> 3x1/1
  w/1 -> 3x1 cross product/1
  3x1 cross product/1 -> Sum/2
  h integrator/1 -> 180 deg/s Max  Gimbal Rate Limiter1/1
  1/h/1 -> To Workspace/1
  det[A]/1 -> Scope2/1
  |h|[A]^-1/1 -> "[A]inv*[hdot]"/1
  Subsystem/1(1/Cond[A]) -> Scope/1, Subsystem3/1(1/Cond[A]), To Workspace4/1

== system Latest_Greatest/CMGs/Subsystem1 ==
  In1 : Inport
  In3 : Inport  Port=2
  In2 : Inport  Port=3
  Displays : Subsystem
      mask Display: disp('Displays')
  Subsystem : Subsystem
      mask Display: disp('DeMux')
  Subsystem2 : Subsystem
      mask Display: disp('CMGs')
  Out1 : Outport  VectorParamsAs1DForOutWhenUnconnected=off
  wires:
  Subsystem/1(Torque) -> Displays/1(Tc), Out1/1
  Subsystem/2(GimbalAngles) -> Displays/2(d)
  In2/1 -> Displays/3(u)
  Subsystem2/1(MP) -> Subsystem/1(SAC/MP)
  In1/1 -> Subsystem2/1(u)
  In3/1 -> Subsystem2/2(gimbal angles)

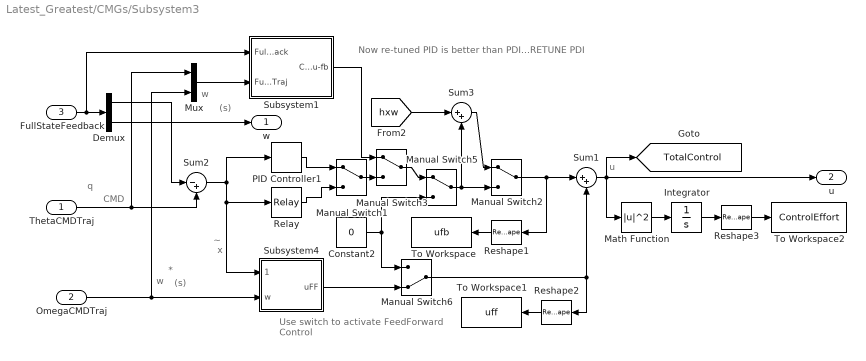
== system Latest_Greatest/CMGs/Subsystem3 ==
  note: u
  note: x
  note: ~
  note: Use switch to activate
      | FeedForward Control
  note: w
  note: (s)
  note: q
  note: CMD
  note: *
  note: (s)
  note: w
  note: Now re-tuned PID is better than PDI...RETUNE PDI
  ThetaCMDTraj : Inport
  OmegaCMDTraj : Inport  Port=2
  FullStateFeedback : Inport  Port=3
  Constant2 : Constant  Value=0
  Demux : Demux  Outputs=2
  Integrator : Integrator
  Manual Switch{1..3,5} (4 alike) : ManualSwitch
  Manual Switch6 : ManualSwitch  CurrentSetting=0
  Math Function : Math  Operator=magnitude^2  SignedPower=on  SaturateOnIntegerOverflow=on
  Mux : Mux  Inputs=2
  PID Controller1 : simulink_need_slupdate/PID Controller  P=-Kpx  I=-Kix  D=-Kdx
  Relay : Relay  OnOutputValue=pi  OffOutputValue=-pi
  Reshape1 : Reshape  OutputDimensions=[1,9]
  Reshape2 : Reshape  OutputDimensions=[1,9]
  Reshape3 : Reshape  OutputDimensions=[1,9]
  Subsystem1 : Subsystem
      mask Display: disp('PDI Controller')
  Subsystem4 : Subsystem
      mask Display: disp('Feedforward')
  Sum1 : Sum  Inputs=|++  SaturateOnIntegerOverflow=on
  Sum2 : Sum  Inputs=|-+  SaturateOnIntegerOverflow=on
  Sum3 : Sum  Inputs=|++  SaturateOnIntegerOverflow=on
  To Workspace : ToWorkspace  VariableName=ufb  SampleTime=-1
  To Workspace1 : ToWorkspace  VariableName=uff  SampleTime=-1
  To Workspace2 : ToWorkspace  VariableName=ControlEffort  SampleTime=-1
  w : Outport  VectorParamsAs1DForOutWhenUnconnected=off
  u : Outport  Port=2  VectorParamsAs1DForOutWhenUnconnected=off
  tag scope: TotalControl=global
  wires:
  Demux/1 -> Sum2/1
  Sum2/1 -> Relay/1, Subsystem4/1(LAMBDA*xtilda), PID Controller1/1
  ThetaCMDTraj/1 -> Sum2/2, Mux/1
  Relay/1 -> Manual Switch1/2
  PID Controller1/1 -> Manual Switch1/1
  Manual Switch1/1 -> Manual Switch3/2
  Demux/2 -> w/1
  Subsystem1/1("Control, u-fb") -> Manual Switch3/1
  FullStateFeedback/1 -> Demux/1, Subsystem1/1(Full State Feedback)
  Sum1/1 -> [TotalControl], u/1, Math Function/1
  Math Function/1 -> Integrator/1
  Integrator/1 -> Reshape3/1
  Reshape1/1 -> To Workspace/1
  Reshape2/1 -> To Workspace1/1
  Reshape3/1 -> To Workspace2/1
  Manual Switch3/1 -> Manual Switch5/1
  Manual Switch6/1 -> Sum1/2, Reshape2/1
  Constant2/1 -> Manual Switch5/2, Manual Switch6/1
  Subsystem4/1(uFF) -> Manual Switch6/2
  Manual Switch5/1 -> Manual Switch2/2, Sum3/2
  Manual Switch2/1 -> Sum1/1, Reshape1/1
  Sum3/1 -> Manual Switch2/1
  [hxw] -> Sum3/1
  OmegaCMDTraj/1 -> Subsystem4/2(w), Mux/2
  Mux/1 -> Subsystem1/2(FullCMDTraj)

== system Latest_Greatest/Subsystem/Subsystem ==
  In1 : Inport
  Demux : Demux  Outputs=3
  To Workspace1 : ToWorkspace  VariableName=roll  SampleTime=-1
  To Workspace2 : ToWorkspace  VariableName=pitch  SampleTime=-1
  To Workspace3 : ToWorkspace  VariableName=yaw  SampleTime=-1
  wires:
  In1/1 -> Demux/1
  Demux/1 -> To Workspace1/1
  Demux/2 -> To Workspace2/1
  Demux/3 -> To Workspace3/1

== system Latest_Greatest/Subsystem2/Tgg ==
  note: Gravity Gradient Torques
  DCM : Inport
  3*mu/Ro^3 : Gain  Gain=3*mu/(h+Re)^3  Multiplication=Matrix(K*u)  SaturateOnIntegerOverflow=on  OutDataTypeStr=Inherit: Same as input  ParamDataTypeStr=Inherit: Same as input
  3x3 cross product : aerospace/Axes Transformations/3x3 cross product
      settings: SourceProductBaseCode=SL
  Jbody : Gain  Gain=Imo  Multiplication=Matrix(K*u)  SaturateOnIntegerOverflow=on  OutDataTypeStr=Inherit: Same as input  ParamDataTypeStr=Inherit: Same as input
  On/Off : Gain  Gain=0  SaturateOnIntegerOverflow=on  OutDataTypeStr=Inherit: Same as input  ParamDataTypeStr=Inherit: Same as input
  Select ci3 : Subsystem
  Tgg : Outport  VectorParamsAs1DForOutWhenUnconnected=off
  wires:
  On/Off/1 -> Tgg/1
  DCM/1 -> Select ci3/1(U)
  Select ci3/1(U(E)) -> Jbody/1, 3x3 cross product/1
  3x3 cross product/1 -> 3*mu/Ro^3/1
  3*mu/Ro^3/1 -> On/Off/1
  Jbody/1 -> 3x3 cross product/2

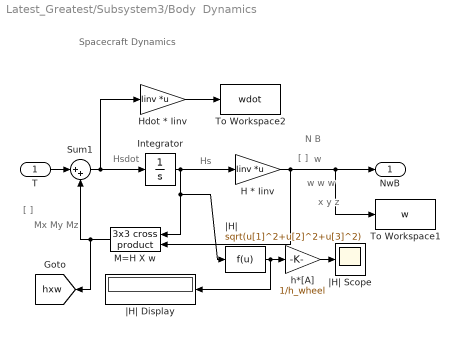
== system Latest_Greatest/Subsystem3/Body  Dynamics ==
  note: w
  note: N B
  note: Hs
  note: Hsdot
  note: [ ]
  note: Mx
      | My
      | Mz
  note: [ ]
  note: w
      | w
      | w
  note: x
      | y
      | z
  note: Spacecraft Dynamics
  T : Inport
  H * Iinv : Gain  Gain=Iinv  Multiplication=Matrix(K*u)  SaturateOnIntegerOverflow=on  OutDataTypeStr=Inherit: Same as input  ParamDataTypeStr=Inherit: Same as input
  Hdot * Iinv : Gain  Gain=Iinv  Multiplication=Matrix(K*u)  SaturateOnIntegerOverflow=on  OutDataTypeStr=Inherit: Same as input  ParamDataTypeStr=Inherit: Same as input
  Integrator : Integrator
  M=H X w : aerospace/Axes Transformations/3x3 cross product
      settings: SourceProductBaseCode=SL
  Sum1 : Sum  Inputs=|++  InputSameDT=on  SaturateOnIntegerOverflow=on  OutDataTypeStr=Inherit: Same as first input
  To Workspace1 : ToWorkspace  VariableName=w  SampleTime=-1
  To Workspace2 : ToWorkspace  VariableName=wdot  SampleTime=-1
  h*[A] : Gain  Gain=1/h_wheel
  |H| : Fcn  Expr=sqrt(u[1]^2+u[2]^2+u[3]^2)
  |H| Display : Display
  |H| Scope : Scope
  NwB : Outport  VectorParamsAs1DForOutWhenUnconnected=off
  tag scope: hxw=global
  wires:
  Integrator/1 -> H * Iinv/1, M=H X w/1, |H|/1
  H * Iinv/1 -> M=H X w/2, NwB/1, To Workspace1/1
  M=H X w/1 -> Sum1/2, [hxw]
  |H|/1 -> |H| Display/1, h*[A]/1
  Sum1/1 -> Integrator/1, Hdot * Iinv/1
  T/1 -> Sum1/1
  h*[A]/1 -> |H| Scope/1
  Hdot * Iinv/1 -> To Workspace2/1

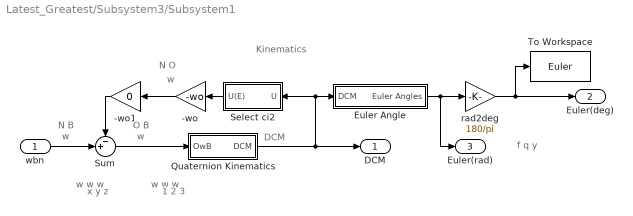
== system Latest_Greatest/Subsystem3/Subsystem1 ==
  note: w
      | w
      | w
  note: x
      | y
      | z
  note: w
  note: N B
  note: w
  note: w
      | w
      | w
  note: 1
      | 2
      | 3
  note: w
  note: O B
  note: DCM
  note: N O
  note: f
      | q
      | y
  note: Kinematics
  wbn : Inport
  -wo : Gain  Gain=-wo  SaturateOnIntegerOverflow=on  OutDataTypeStr=Inherit: Same as input  ParamDataTypeStr=Inherit: Same as input
  -wo1 : Gain  Gain=0  SaturateOnIntegerOverflow=on  OutDataTypeStr=Inherit: Same as input  ParamDataTypeStr=Inherit: Same as input
  Euler Angle : Subsystem
  Quaternion Kinematics : Subsystem
  Select ci2 : Subsystem
  Sum : Sum  Inputs=-+|  InputSameDT=on  SaturateOnIntegerOverflow=on  OutDataTypeStr=Inherit: Same as first input
  To Workspace : ToWorkspace  VariableName=Euler  SampleTime=-1
  rad2deg : Gain  Gain=180/pi  SaturateOnIntegerOverflow=on  OutDataTypeStr=Inherit: Same as input  ParamDataTypeStr=Inherit: Same as input
  DCM : Outport  VectorParamsAs1DForOutWhenUnconnected=off
  Euler(deg) : Outport  Port=2  VectorParamsAs1DForOutWhenUnconnected=off
  Euler(rad) : Outport  Port=3  VectorParamsAs1DForOutWhenUnconnected=off
  wires:
  Sum/1 -> Quaternion Kinematics/1(OwB)
  -wo/1 -> -wo1/1
  Select ci2/1(U(E)) -> -wo/1
  Quaternion Kinematics/1(DCM) -> Select ci2/1(U), Euler Angle/1(DCM), DCM/1
  -wo1/1 -> Sum/1
  wbn/1 -> Sum/2
  Euler Angle/1(Euler Angles) -> rad2deg/1, Euler(rad)/1
  rad2deg/1 -> Euler(deg)/1, To Workspace/1

== system Latest_Greatest/Subsystem5/OBSERVERS (MASK THIS SUBSYSTEM AS CLASS DEMO)1 ==
  Full State Feedback : Inport
  Demux : Demux  Outputs=2
  Subsystem : Subsystem
      mask Display: disp('Luenberger & PID Observers')
  Terminator : Terminator
  Estimated full state feedback (Euler-rad) : Outport  VectorParamsAs1DForOutWhenUnconnected=off
  wires:
  Demux/1 -> Subsystem/1(Euler Angle (rad))
  Demux/2 -> Terminator/1
  Subsystem/1(Estimated Full  State Feedback) -> Estimated full state feedback (Euler-rad)/1
  Full State Feedback/1 -> Demux/1

== system Latest_Greatest/Subsystem5/Subsystem2 ==
  note: Noisy Sensor
  Full State Feedback : Inport
  Random Number : RandomNumber  Variance=NoiseVariance  SampleTime=0
  Sum1 : Sum  Inputs=|++
  Noisy  State Feedback : Outport  VectorParamsAs1DForOutWhenUnconnected=off
  wires:
  Random Number/1 -> Sum1/2
  Sum1/1 -> Noisy  State Feedback/1
  Full State Feedback/1 -> Sum1/1

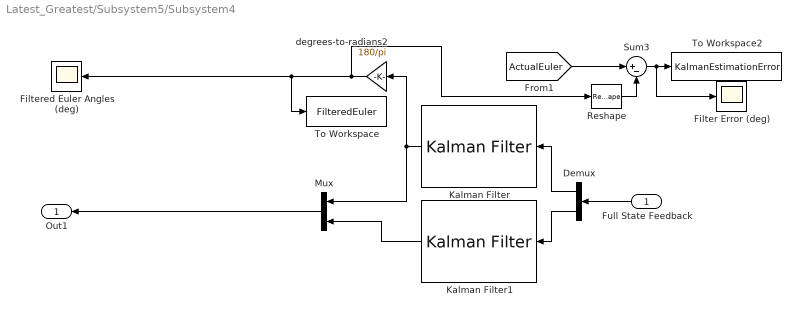
== system Latest_Greatest/Subsystem5/Subsystem4 ==
  Full State Feedback : Inport
  Demux : Demux  Outputs=2
  Filter Error (deg) : Scope
      settings: StopFcn=|
      | %Simulink figure properties
      | shh=get(0,'ShowHiddenHandles');
      | set(0,'ShowHiddenHandles','On')
      | set(gcf,'menubar','figure')
      | set(gcf,'CloseRequestFcn','closereq')
      | set(gcf,'DefaultLineClipping','Off')
      | set(0,'ShowHiddenHandles',shh)
  Filtered Euler Angles (deg) : Scope
      settings: StopFcn=|
      | %Simulink figure properties
      | shh=get(0,'ShowHiddenHandles');
      | set(0,'ShowHiddenHandles','On')
      | set(gcf,'menubar','figure')
      | set(gcf,'CloseRequestFcn','closereq')
      | set(gcf,'DefaultLineClipping','Off')
      | set(0,'ShowHiddenHandles',shh)
  Kalman Filter : dspadpt3/Kalman Filter  num_targets=1  sourceEnable=Always  isReset=on  X=zeros([3, 1])  P=10*eye(3)  A=eye(3)  sourceMeasure=Specify via Dialog  H=eye(3)  Q=0.05*eye(3)  R=eye(3)  isOutputEstMeasure=off  isOutputEstState=on  isOutputEstError=off  isOutputPrdMeasure=off  isOutputPrdState=off  isOutputPrdError=off
      settings: SourceProductBaseCode=DS
  Kalman Filter1 : dspadpt3/Kalman Filter  num_targets=1  sourceEnable=Always  isReset=on  X=zeros([3, 1])  P=10*eye(3)  A=eye(3)  sourceMeasure=Specify via Dialog  H=eye(3)  Q=0.05*eye(3)  R=eye(3)  isOutputEstMeasure=off  isOutputEstState=on  isOutputEstError=off  isOutputPrdMeasure=off  isOutputPrdState=off  isOutputPrdError=off
      settings: SourceProductBaseCode=DS
  Mux : Mux  Inputs=2
  Reshape : Reshape
  Sum3 : Sum  Inputs=|+-
  To Workspace : ToWorkspace  VariableName=FilteredEuler  SampleTime=-1
  To Workspace2 : ToWorkspace  VariableName=KalmanEstimationError  SampleTime=-1
  degrees-to-radians2 : Gain  Gain=180/pi
  Out1 : Outport  VectorParamsAs1DForOutWhenUnconnected=off
  wires:
  [ActualEuler] -> Sum3/1
  Reshape/1 -> Sum3/2
  Sum3/1 -> Filter Error (deg)/1, To Workspace2/1
  degrees-to-radians2/1 -> Reshape/1, Filtered Euler Angles (deg)/1, To Workspace/1
  Kalman Filter/1 -> degrees-to-radians2/1, Mux/1
  Demux/2 -> Kalman Filter1/1
  Full State Feedback/1 -> Demux/1
  Demux/1 -> Kalman Filter/1
  Mux/1 -> Out1/1
  Kalman Filter1/1 -> Mux/2

== system Latest_Greatest/Subsystem5/Subsystem5 ==
  note: See Bong Wie
      | Generalized Second Order Filters
      | 2nd Edition pg 137
  u : Inport
  Demux : Demux  Outputs=6
  Mux : Mux  Inputs=6
  Transfer Fcn{,1..5} (6 alike) : TransferFcn  Numerator="[1/wz^2   2*dampZ/wz  1]"  Denominator="[1/wp^2   2*dampP/wp  1]"
  u(filtered) : Outport  VectorParamsAs1DForOutWhenUnconnected=off
  wires:
  Mux/1 -> u(filtered)/1
  u/1 -> Demux/1
  Transfer Fcn/1 -> Mux/1
  Transfer Fcn1/1 -> Mux/2
  Transfer Fcn2/1 -> Mux/3
  Transfer Fcn3/1 -> Mux/4
  Transfer Fcn4/1 -> Mux/5
  Transfer Fcn5/1 -> Mux/6
  Demux/1 -> Transfer Fcn/1
  Demux/2 -> Transfer Fcn1/1
  Demux/3 -> Transfer Fcn2/1
  Demux/4 -> Transfer Fcn3/1
  Demux/5 -> Transfer Fcn4/1
  Demux/6 -> Transfer Fcn5/1

== system Latest_Greatest/CMGs/CMG Steering Logic1/Subsystem ==
  "[A]" : Inport
  Divide : Product  Inputs=/*
  max (SVD[A]) : MATLABFcn  MATLABFcn=max(svd(u))
  min (SVD[A]) : MATLABFcn  MATLABFcn=min(svd(u))
  1/Cond[A] : Outport  VectorParamsAs1DForOutWhenUnconnected=off
  wires:
  Divide/1 -> 1/Cond[A]/1
  max (SVD[A])/1 -> Divide/2
  min (SVD[A])/1 -> Divide/1
  "[A]"/1 -> max (SVD[A])/1, min (SVD[A])/1

== system Latest_Greatest/CMGs/CMG Steering Logic1/Subsystem1 ==
  delta : Inport
  3x4 : Reshape  OutputDimensionality=Customize  OutputDimensions=[3,4]
  "[A] Matrix" : MATLABFcn  MATLABFcn="[ -cos(beta(1))*cos(u(1)),  sin(u(2)), cos(beta(3))*cos(u(3)), 0   ;  -sin(u(1)),  -cos(beta(2))*cos(u(2)),  sin(u(3)),   0;  sin(beta(1))*cos(u(1)),  sin(beta(2))*cos(u(2)),  sin(beta(3))*cos(u(3)),   0  ]"
  "[A]" : Outport  VectorParamsAs1DForOutWhenUnconnected=off
  wires:
  "[A] Matrix"/1 -> 3x4/1
  delta/1 -> "[A] Matrix"/1
  3x4/1 -> "[A]"/1

== system Latest_Greatest/CMGs/CMG Steering Logic1/Subsystem3 ==
  1/Cond[A] : Inport
  deltaDot : Inport  Port=2
  Switch : Switch  Threshold=2.21
  Unit Delay : UnitDelay  SampleTime=-1  HasFrameUpgradeWarning=on
  Out1 : Outport  VectorParamsAs1DForOutWhenUnconnected=off
  wires:
  1/Cond[A]/1 -> Switch/2
  deltaDot/1 -> Switch/1
  Switch/1 -> Unit Delay/1, Out1/1
  Unit Delay/1 -> Switch/3

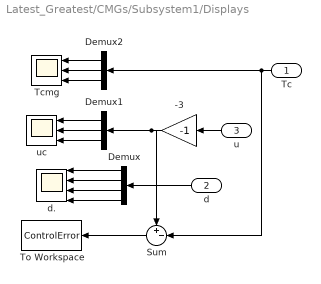
== system Latest_Greatest/CMGs/Subsystem1/Displays ==
  Tc : Inport
  d : Inport  Port=2
  u : Inport  Port=3
  -3 : Gain  Gain=-1  SaturateOnIntegerOverflow=on  OutDataTypeStr=Inherit: Same as input  ParamDataTypeStr=Inherit: Same as input
  Demux : Demux
  Demux1 : Demux  Outputs=3
  Demux2 : Demux  Outputs=3
  Sum : Sum  Inputs=+-|
  Tcmg : Scope  NumInputPorts=3
  To Workspace : ToWorkspace  VariableName=ControlError  SampleTime=-1
  d. : Scope  NumInputPorts=4
  uc : Scope  NumInputPorts=3
  wires:
  d/1 -> Demux/1
  u/1 -> -3/1
  Demux/4 -> d./4
  Demux/3 -> d./3
  Demux/2 -> d./2
  Demux/1 -> d./1
  -3/1 -> Demux1/1, Sum/1
  Tc/1 -> Demux2/1, Sum/2
  Demux2/1 -> Tcmg/1
  Demux2/2 -> Tcmg/2
  Demux2/3 -> Tcmg/3
  Demux1/1 -> uc/1
  Demux1/2 -> uc/2
  Demux1/3 -> uc/3
  Sum/1 -> To Workspace/1

== system Latest_Greatest/CMGs/Subsystem1/Subsystem ==
  SAC/MP : Inport
  Demux : Demux  Outputs=8
  Mux : Mux  Inputs=3
  Mux1 : Mux
  To Workspace : ToWorkspace  VariableName=flag  SampleTime=-1
  Torque : Outport  VectorParamsAs1DForOutWhenUnconnected=off
  GimbalAngles : Outport  Port=2  VectorParamsAs1DForOutWhenUnconnected=off
  wires:
  SAC/MP/1 -> Demux/1
  Demux/8 -> To Workspace/1
  Demux/1 -> Mux/1
  Demux/2 -> Mux/2
  Demux/3 -> Mux/3
  Demux/4 -> Mux1/1
  Demux/5 -> Mux1/2
  Demux/6 -> Mux1/3
  Demux/7 -> Mux1/4
  Mux1/1 -> GimbalAngles/1
  Mux/1 -> Torque/1

== system Latest_Greatest/CMGs/Subsystem1/Subsystem2 ==
  note: Gimbal Angles
  note: u
  note: flag
  u : Inport
  gimbal angles : Inport  Port=2
  Constant1 : Constant
  Mux1 : Mux  Inputs=3
  MP : Outport  VectorParamsAs1DForOutWhenUnconnected=off
  wires:
  u/1 -> Mux1/1
  Constant1/1 -> Mux1/3
  Mux1/1 -> MP/1
  gimbal angles/1 -> Mux1/2

== system Latest_Greatest/CMGs/Subsystem3/Subsystem1 ==
  note: e(s)
  note: w
  note: (s)
  note: q
  note: (s)
  note: u(s)
  note: *
  note: q
  note: (s)
  note: w
  note: *
  note: (s)
  Full State Feedback : Inport
  FullCMDTraj : Inport  Port=2
  Demux : Demux  Outputs=2
  Demux1 : Demux  Outputs=2
  Integrator9 : Integrator
  Subsystem25 : Subsystem
      mask Display: disp('Ki')
  Subsystem26 : Subsystem
      mask Display: disp('Kp')
  Subsystem27 : Subsystem
      mask Display: disp('Kd')
  Sum12 : Sum  Inputs=|+-
  Sum14 : Sum  Inputs=+++
  Sum15 : Sum  Inputs=|+-
  "Control, u-fb" : Outport  VectorParamsAs1DForOutWhenUnconnected=off
  wires:
  Sum14/1 -> "Control, u-fb"/1
  Demux/1 -> Sum12/2
  Sum15/1 -> Subsystem27/1(In1)
  Integrator9/1 -> Subsystem25/1(In1)
  Sum12/1 -> Subsystem26/1(In1), Integrator9/1
  Subsystem27/1(Out1) -> Sum14/3
  Subsystem26/1(Out1) -> Sum14/2
  Subsystem25/1(Out1) -> Sum14/1
  Demux1/2 -> Sum15/1
  Demux1/1 -> Sum12/1
  Full State Feedback/1 -> Demux/1
  Demux/2 -> Sum15/2
  FullCMDTraj/1 -> Demux1/1
